simulink model "TB_6DOF_v1"  (R2026a)
settings: Solver=ode45  MaxStep=0.001
PreLoadFcn:
  | mc_inputs
settings Model: Creator=aditi  LastModifiedBy=aditi

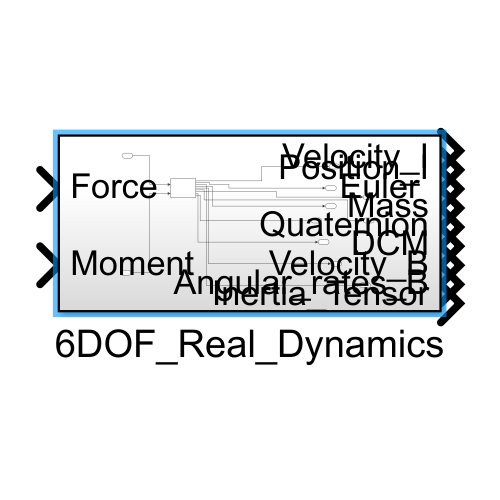
[thumbnail: Simulink's stored preview of the top-level diagram]
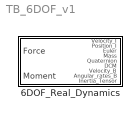
== system TB_6DOF_v1 ==
  6DOF_Real_Dynamics : Subsystem

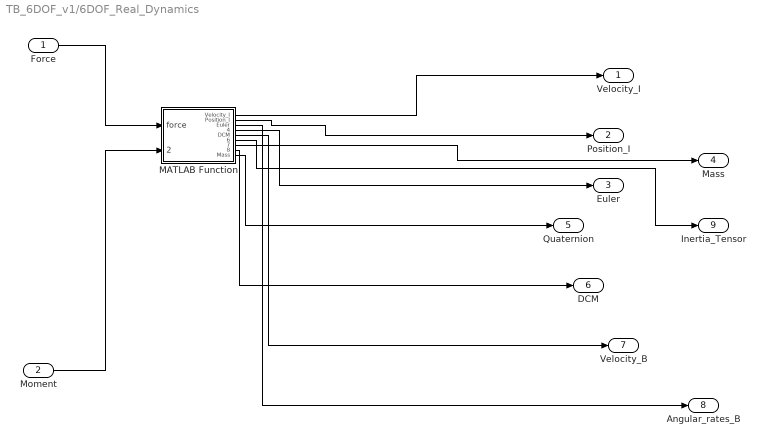
== system TB_6DOF_v1/6DOF_Real_Dynamics ==
  Force : Inport
  Moment : Inport  Port=2
  MATLAB Function : MATLAB Function  TreatAsAtomicUnit=on
  Velocity_I : Outport
  Position_I : Outport  Port=2
  "Euler " : Outport  Port=3
  Mass : Outport  Port=4
  Quaternion : Outport  Port=5
  DCM : Outport  Port=6
  Velocity_B : Outport  Port=7
  Angular_rates_B : Outport  Port=8
  Inertia_Tensor : Outport  Port=9
  wires:
  Moment/1 -> MATLAB Function/2(moment)
  Force/1 -> MATLAB Function/1(force)
  MATLAB Function/1(Velocity_I) -> Velocity_I/1
  MATLAB Function/2(Position_I) -> Position_I/1
  MATLAB Function/4(Quaternion) -> "Euler "/1
  MATLAB Function/7(Angular_rates_B) -> Mass/1
  MATLAB Function/6(Velocity_B) -> Inertia_Tensor/1
  MATLAB Function/9(Mass) -> Quaternion/1
  MATLAB Function/8(Inertia_Tensor) -> DCM/1
  MATLAB Function/5(DCM) -> Velocity_B/1
  MATLAB Function/3(Euler) -> Angular_rates_B/1

== matlab function TB_6DOF_v1/6DOF_Real_Dynamics/MATLAB Function ==
  data: Velocity_I output; force input; moment input; Position_I output; Euler output; Quaternion output; DCM output; Velocity_B output; Angular_rates_B output; Inertia_Tensor output; Mass output
function [Velocity_I, Position_I, Euler, Quaternion, DCM, Velocity_B, Angular_rates_B, Inertia_Tensor, Mass] = custom_aerospace_6dof(force, moment)
    % =====================================================================
    % ALL 9 OUTPUTS DERIVED DIRECTLY FROM FIRST-PRINCIPLES PHYSICS
    % =====================================================================
    
    %% 1. TIME STEP & MASS DECAY PARAMETERS
    dt     = 0.01;                 % Time step size (seconds)
    m_dot  = -0.5;                 % Mass loss rate (kg/s)
    
    %% 2. PERSISTENT STATE MEMORY
    persistent m_state V_b_state omega_b_state q_state P_i_state
    
    if isempty(m_state)
        m_state       = 500.0;     % Initial Mass (kg)
        V_b_state     = [0;0;0];   % Initial Body Velocity [u; v; w]
        omega_b_state = [0;0;0];   % Initial Body Angular Rates [p; q; r]
        q_state       = [1;0;0;0]; % Initial Quaternion (Aligned with ground)
        P_i_state     = [0;0;0];   % Initial Inertial Position [x; y; z]
    end

    %% 3. MASS & INERTIA TENSOR CALCULATION
    % Update mass and map directly to output
    m_state = m_state + m_dot * dt;
    Mass = m_state; 
    
    % Track changing base inertia shape profile as fuel drains
    I_tank = diag([100, 250, 250]) + diag([0.1, 0.2, 0.2]) * (500 - Mass); 
    I_dot  = diag([-0.1, -0.2, -0.2]); 
    
    % Calculate shifting Center of Gravity displacement [xd; yd; zd]
    % Apply subtractive Parallel Axis Theorem matrix to find inertia around the real CG
    x_d = 0.05 * (500 - Mass); 
    Inertia_Tensor = I_tank - Mass * [0,    0,    0;
                                      0,  x_d^2,  0;
                                      0,    0,  x_d^2];

    %% 4. ROTATIONAL DYNAMICS (Angular Rates)
    % Derived via Euler's Rotational Equations + Variable Inertia Correction
    omega_b_dot = Inertia_Tensor \ (moment - cross(omega_b_state, Inertia_Tensor * omega_b_state) - I_dot * omega_b_state);
    omega_b_state = omega_b_state + omega_b_dot * dt;
    Angular_rates_B = omega_b_state; % Map to output

    %% 5. TRANSLATIONAL DYNAMICS (Body Velocity)
    % Derived via Newton's Second Law + Coriolis/Transport Theorem
    V_b_dot = (force / Mass) - (m_dot / Mass) * V_b_state - cross(Angular_rates_B, V_b_state);
    V_b_state = V_b_state + V_b_dot * dt;
    Velocity_B = V_b_state; % Map to output

    %% 6. ORIENTATION KINEMATICS (Quaternion & DCM)
    % Quaternion derivative via 4D skew-symmetric matrix multiplication
    p = Angular_rates_B(1); q_val = Angular_rates_B(2); r = Angular_rates_B(3);
    Omega_q = [0,  -p, -q_val, -r;
               p,   0,   r, -q_val;
               q_val, -r,   0,   p;
               r,   q_val, -p,   0];
    q_dot = 0.5 * Omega_q * q_state;
    
    % Integrate and strictly normalize to prevent numerical axis warping
    q_state = q_state + q_dot * dt;
    q_state = q_state / norm(q_state);
    Quaternion = q_state; % Map to output 
    
    % Construct DCM directly from Quaternion components (Rodrigues derivation)
  
    q0 = Quaternion(1); q1 = Quaternion(2); q2 = Quaternion(3); q3 = Quaternion(4);
    DCM = [1 - 2*(q2^2 + q3^2),   2*(q1*q2 - q0*q3),   2*(q1*q3 + q0*q2);
           2*(q1*q2 + q0*q3), 1 - 2*(q1^2 + q3^2),   2*(q2*q3 - q0*q1);
           2*(q1*q3 - q0*q2), 2*(q2*q3 + q0*q1), 1 - 2*(q1^2 + q2^2)];

    %% 7. BRIDGING KINEMATICS TO INERTIAL SPACE (Inertial Velocity & Position)
    % Rotate body velocity to inertial velocity via DCM matrix multiplication
    Velocity_I = DCM * Velocity_B; 
    
    % Pure linear integration for Inertial Position
    P_i_state = P_i_state + Velocity_I * dt;
    Position_I = P_i_state; % Map to output

    %% 8. EULER ANGLES EXTRACTION
    phi   = atan2(DCM(3,2), DCM(3,3));     % Roll
    theta = -asin(DCM(3,1));              % Pitch
    psi   = atan2(DCM(2,1), DCM(1,1));     % Yaw
    Euler = [phi; theta; psi];            % Map to output
end
